simulink model "at3_2"  (R2020a)
settings: Solver=VariableStepAuto  StartTime=0.0  StopTime=3.5  RelTol=1e-3
model workspace (MAT data in the model file):
  T = [1 0 0 0 0 1 0 0 0 0 1 0 ... (16 elements, 4x4)]
  bd = 5
  kd = 10
  md = 1
  myFd = [0; 0; 5; 0; 0; 0]
  mybot : SerialLink (value not decoded)
values from neighbouring files (symbols this model uses):
  Fd2 = [0 0 5 0 0 0]'    [main.m]
  Fd3 = [0 0 0 0 0 0]'    [main.m]
  m = [171.459 140.993 94.498 31.976 31.091 0.606]    [I.mat]    (also in main.m = [205.811,102.832,267.675,25.069,10.895,3.354]; maincircle.m = [205.811,102.832,267.675,25.069,10.895,3.354])
undefined symbols (not defined in the file or in its folder): X, Y, Z
libraries: sm_lib x76, nesl_utility x31, simulink_extras x21, roblocks x16, simulink x7
(part 3 of 3)

== matlab function at3_2/MATLAB Function ==
  data: hole input; T input; Fe output; v input; state input
function Fe = mysensor(hole,T,v,state)
% 由末端的齐次变换矩阵以及孔的位置计算得到力
% 正常情况下n为（0，0，-1）,轴为d=0.01，孔D=0.03
pos=T(1:3,4);
n=-T(1:3,3);
Fe=zeros(6,1);
miu=0.3;
d1=0.01;d2=0.03;E=210e9;
l=0.3*n;
v=v(1:2);
% 重要比例参数
mycoef=[1e-4,1e-3,1e-3];
d=norm(pos(1:2)-hole(1:2));

%分为三种情况来计算力，轴孔不接触，轴孔接触，轴孔配合
S1=pi/4*d1^2; S2=pi/4*d2^2;
if state==1
    Fe=zeros(6,1);
elseif state==2
%（1）轴孔不接触
    % 简单版本
    if d>(d1+d2)/2
        delta_z=pos(3)-hole(3);
        if delta_z>=0
            Fe(3)=0;
        else
            Fe(3)=-E*delta_z*S1;
        end
        if norm(v)==0
            Fe(1)=0;
            Fe(2)=0;
        else
            Fe(1)=-miu*Fe(3)*v(1)/norm(v);
            Fe(2)=-miu*Fe(3)*v(2)/norm(v);
        end

        Fe(4)=Fe(2)*l(3)-Fe(3)*l(2);
        Fe(5)=Fe(3)*l(1)-Fe(1)*l(3);
        Fe(6)=Fe(1)*l(2)-Fe(2)*l(1);
        Fe=Fe*mycoef(1);
    else
    %（2）轴孔接触
        r1=d1/2;r2=d2/2;
        ang=zeros(2);
        if abs((r2^2+d^2-r1^2)/(2*r2*d))>1
            hhhh=[(r1^2+d^2-r2^2)/(2*r1*d),(r2^2+d^2-r1^2)/(2*r2*d)]
            d
        end
        ang(1)=acos((r1^2+d^2-r2^2)/(2*r1*d));
        ang(2)=acos((r2^2+d^2-r1^2)/(2*r2*d));
        S=ang(1)*r1^2+ang(2)*r2^2-r1*d*sin(ang(1));

        delta_z=pos(3)-hole(3);
        if delta_z>=0
            Fe(3)=0;
        else
            Fe(3)=-E*delta_z*S;
        end

        if norm(v)==0
            Fe(1)=0;
            Fe(2)=0;
        else
            Fe(1)=-miu*Fe(3)*v(1)/norm(v);
            Fe(2)=-miu*Fe(3)*v(2)/norm(v);
        end

        Fe(4)=Fe(2)*l(3)-Fe(3)*l(2);
        Fe(5)=Fe(3)*l(1)-Fe(1)*l(3);
        Fe(6)=Fe(1)*l(2)-Fe(2)*l(1);
        Fe=Fe*mycoef(2);
    end
else
%（3）轴孔配合
    temp=(hole(3)-pos(3))/n(3);
    x1=temp*n(1)+pos(1);
    y1=temp*n(2)+pos(2);
    
    EE=1;
    d=norm([x1;y1]-hole(1:2))-0.01;
    if d<0
        Fe=zeros(6,1);
    else
        nn=n(1:2);
        Fe(1)=-EE*d/d1*nn(1)/norm(nn);
        Fe(2)=-EE*d/d1*nn(2)/norm(nn);
        Fe(3)=miu*EE*d/d1;
        
        %作用力从沿边开始作用
        l=l-temp*n;
        Fe(4)=Fe(2)*l(3)-Fe(3)*l(2);
        Fe(5)=Fe(3)*l(1)-Fe(1)*l(3);
        Fe(6)=Fe(1)*l(2)-Fe(2)*l(1);
        Fe=Fe*mycoef(3);
    end
end

end

== matlab function at3_2/Admittance_Control/MATLAB Function ==
  data: xe input; dxe input; MDK input; Fe input; ddxe output
function ddxe = admit(xe,dxe,MDK,Fe)
%导纳控制器计算
M=MDK(1)*eye(6);
D=MDK(2)*eye(6);
K=MDK(3)*eye(6);

ddxe=M\(Fe-D*dxe-K*xe)

end

== matlab function at3_2/Admittance_Control/MATLAB Function3 ==
  data: state input; S output
function S = myswitch(state)
% state(1.下降阶段 2.寻孔阶段 3.插孔阶段)
% thresh 各个阶段的节点时间
S=zeros(6);

if state==1
    S=zeros(6);
elseif state==2
    S=zeros(6);
    S(3,3)=1;
else
    S=eye(6);
end

end

== matlab function at3_2/Pos_control/Robot System1/MATLAB Function ==
  data: Tr input; rpy output
function rpy = Tr2rpy_xyz(Tr)
R=Tr;
rpy=zeros(1,3);

if abs(abs(R(1,3)) - 1) < eps  % when |R13| == 1
    % singularity
    rpy(1) = 0;  % roll is zero
    if R(1,3) > 0
    rpy(3) = atan2( R(3,2), R(2,2));   % R+Y
    else
         rpy(3) = -atan2( R(2,1), R(3,1));   % R-Y
    end
    rpy(2) = asin(R(1,3));
else
    rpy(1) = -atan2(R(1,2), R(1,1));
    rpy(3) = -atan2(R(2,3), R(3,3));
    [~,k] = max(abs( [R(1,1) R(1,2) R(2,3) R(3,3)] ));
    switch k
        case 1
            rpy(2) =  atan(R(1,3)*cos(rpy(1))/R(1,1));
        case 2
            rpy(2) = -atan(R(1,3)*sin(rpy(1))/R(1,2));
        case 3
            rpy(2) = -atan(R(1,3)*sin(rpy(3))/R(2,3));
        case 4
            rpy(2) =  atan(R(1,3)*cos(rpy(3))/R(3,3));
    end
end

rpy=rpy*180/pi;

end

== matlab function at3_2/Pos_control/Robot System1/MATLAB Function1 ==
  data: R input; xyz input; T output
function T = transf(R,xyz)

T=eye(4);
T(1:3,1:3)=R;
T(1:3,4)=-xyz';
%z方向偏置
T(3,4)=T(3,4)-0.23333
end

== matlab function at3_2/Admittance_Control/Subsystem/MATLAB Function1 ==
  data: T input; mytheta output; start input
function mytheta = inverse_kinematics(T,start)
%计算逆运动学求解,输入末端齐次变换矩阵及起始角度，输出唯一解。
%推导过程见word。

T(abs(T)<1e-4) = 0 ;

%D-H参数
d1 = 0.29333;
d4 = 0.87133;
d6 = 0.10667+0.3;
a1 = 266.67/1000;
a2 = 2/3;

qlim = zeros(6,2);
qlim(1,:)=[-pi,pi];
qlim(2,:)=[-71.48/180*pi,73.52/180*pi];
qlim(3,:)=[-204.22/180*pi,65.78/180*pi];
qlim(4,:)=[-pi,pi];
qlim(5,:)=[-110/180*pi,110/180*pi];
qlim(6,:)=[-pi,pi];

theta=zeros(8,6);
theta1=zeros(4,1);
theta2=zeros(4,1);
theta3=zeros(4,1);
R36=zeros(3,3,4);

%第一步
p06=T(1:3,4);
R06=T(1:3,1:3);
pw=p06-R06*[0 0 d6]';
pwx=pw(1);
pwy=pw(2);
pwz=pw(3);

%第二步
theta1(1)=atan2(pwy,pwx);
theta1(2)=theta1(1);
theta1(3)=theta1(1);
theta1(4)=theta1(3);
s3=( a2^2+d4^2-(pwx-a1*cos(theta1(1)))^2+(pwy-a1*sin(theta1(1)))^2-(pwz-d1)^2 )/2/d4/a2;
if abs(s3)>1
    p06
    R06*[0 0 d6]'
    pw
    T
    s3
    fprintf('s3 error!\n');
end
c3_1=sqrt(1-s3^2);
c3_2=-c3_1;
theta3(1)=atan2(s3,c3_1);
theta3(2)=theta3(1);
theta3(3)=atan2(s3,c3_2);
theta3(4)=theta3(3);

%theta2的解，其中1，2，3，4与theta3一一对应
% c2_1=( sqrt(pwx^2+pwy^2)*(a2-d4*s3)-(pwz-d1)*d4*c3_1 )/( a2^2+d4^2-2*a2*d4*s3 );
% s2_1=( -(pwz-d1)*(a2-d4*s3)-sqrt(pwx^2+pwy^2)*d4*c3_1 )/( a2^2+d4^2-2*a2*d4*s3 );
% theta2(1)=atan2(s2_1,c2_1);
% c2_2=( sqrt(pwx^2+pwy^2)*(a2-d4*s3)-(pwz-d1)*d4*c3_2)/( a2^2+d4^2-2*a2*d4*s3 );
% s2_2=( -(pwz-d1)*(a2-d4*s3)-sqrt(pwx^2+pwy^2)*d4*c3_2 )/( a2^2+d4^2-2*a2*d4*s3 );
% theta2(2)=atan2(s2_2,c2_2);
% c2_3=( -sqrt(pwx^2+pwy^2)*(a2-d4*s3)-(pwz-d1)*d4*c3_1 )/( a2^2+d4^2-2*a2*d4*s3 );
% s2_3=( -(pwz-d1)*(a2-d4*s3)+sqrt(pwx^2+pwy^2)*d4*c3_1 )/( a2^2+d4^2-2*a2*d4*s3 );
% theta2(3)=atan2(s2_3,c2_3);
% c2_4=( -sqrt(pwx^2+pwy^2)*(a2-d4*s3)-(pwz-d1)*d4*c3_2)/( a2^2+d4^2-2*a2*d4*s3 );
% s2_4=( -(pwz-d1)*(a2-d4*s3)+sqrt(pwx^2+pwy^2)*d4*c3_2 )/( a2^2+d4^2-2*a2*d4*s3 );
% theta2(4)=atan2(s2_4,c2_4);

for i=[1,3]
aa=pwz-d1-cos(theta3(i))*d4;
bb=2*a2-2*sin(theta3(i))*d4;
cc=pwz-d1+cos(theta3(i))*d4;
% theta2(1)=2*atan2(-bb-sqrt(bb^2-4*aa*cc),2*aa)
if bb^2-4*aa*cc<0
    bb^2-4*aa*cc
    fprintf('deta error\n!');
end
theta2(i)=2*atan((-bb-sqrt(bb^2-4*aa*cc))/(2*aa))+pi/2;
theta2(i+1)=2*atan((-bb+sqrt(bb^2-4*aa*cc))/(2*aa))+pi/2;

end

theta1(1)=atan2(pwy,pwx);
%theta1(2)=atan2(-pwy,-pwx);
theta1(2)=-atan2(pwy,pwx);
theta1(3)=atan2(pwy,pwx);
%theta1(4)=atan2(-pwy,-pwx);
theta1(4)=-atan2(pwy,pwx);

%第三步、四
R03_1=[sin(theta2(1)+theta3(1))*cos(theta1(1)) sin(theta1(1)) cos(theta2(1)+theta3(1))*cos(theta1(1));...
    sin(theta2(1)+theta3(1))*sin(theta1(1)) -cos(theta1(1)) cos(theta2(1)+theta3(1))*sin(theta1(1));...
    cos(theta2(1)+theta3(1)) 0 -sin(theta2(1)+theta3(1)) ];
R36(:,:,1)=inv(R03_1)*R06;
R03_2=[sin(theta2(2)+theta3(2))*cos(theta1(2)) sin(theta1(2)) cos(theta2(2)+theta3(2))*cos(theta1(2));...
    sin(theta2(2)+theta3(2))*sin(theta1(2)) -cos(theta1(2)) cos(theta2(2)+theta3(2))*sin(theta1(2));...
    cos(theta2(2)+theta3(2)) 0 -sin(theta2(2)+theta3(2))];
R36(:,:,2)=inv(R03_2)*R06;
R03_3=[sin(theta2(3)+theta3(3))*cos(theta1(3)) sin(theta1(3)) cos(theta2(3)+theta3(3))*cos(theta1(3));...
    sin(theta2(3)+theta3(3))*sin(theta1(3)) -cos(theta1(3)) cos(theta2(3)+theta3(3))*sin(theta1(3));...
    cos(theta2(3)+theta3(3)) 0 -sin(theta2(3)+theta3(3))];
R36(:,:,3)=inv(R03_3)*R06;
R03_4=[sin(theta2(4)+theta3(4))*cos(theta1(4)) sin(theta1(4)) cos(theta2(4)+theta3(4))*cos(theta1(4));...
    sin(theta2(4)+theta3(4))*sin(theta1(4)) -cos(theta1(4)) cos(theta2(4)+theta3(4))*sin(theta1(4));...
    cos(theta2(4)+theta3(4)) 0 -sin(theta2(4)+theta3(4))];
R36(:,:,4)=inv(R03_4)*R06;

%第五步
n=1;
for i=1:4
    R=R36(:,:,i);
    a3x=R(1,3);
    a3y=R(2,3);
    a3z=R(3,3);
    s3z=R(3,2);
    n3z=R(3,1);
    
    theta4_1=atan2(-a3y,-a3x);
    theta5_1=atan2(sqrt(a3x^2+a3y^2),a3z);
    theta6_1=atan2(-s3z,n3z);
    theta4_2=atan2(a3y,a3x);
    theta5_2=atan2(-sqrt(a3x^2+a3y^2),a3z);
    theta6_2=atan2(s3z,-n3z);
    
    %输出结果
    % theta(n,:)=[theta1(i) theta2(i)-pi/2 theta3(i) theta4_1 theta5_1 theta6_1];
    theta(n,:)=[theta1(i) theta2(i) theta3(i) theta4_1 theta5_1 theta6_1];
    n=n+1;
    % theta(n,:)=[theta1(i) theta2(i)-pi/2 theta3(i) theta4_2 theta5_2 theta6_2];
    theta(n,:)=[theta1(i) theta2(i) theta3(i) theta4_2 theta5_2 theta6_2];
    n=n+1;
end

%根据关节角度取舍
k = [];
for i = 1:8
    flag = 0;
    for j = 1:6
        if theta(i,j)<qlim(j,1)||theta(i,j)>qlim(j,2)
            flag = 1;
        end
    end
    % flag=0表示这个解对
    
    if ~flag
        k = [k,i];
    end
end
%无解情况
q=zeros(1,6);
if isempty(k)
    q = zeros(1,6);
else
    
theta_kexing = theta(k,:);

%逆解唯一性约束条件
w = [1 1 1 3 3 3];
min_los = 100;
for i = 1:size(theta_kexing,1)
    p = pos(theta_kexing);
    % p_start = pos(start);
    los = 0;
    for j = 1:6
        los = los + w(j)*abs(theta_kexing(i,j)-start(j))*norm(p(:,j)-p(:,j));
    end
        if los<min_los
            q = theta_kexing(i,:);
            min_los = los;
        end
end
end

mytheta=q';

end
